simulink model "continuous_ex"  (R2022b)
settings: Solver=VariableStepAuto  StartTime=0.0  StopTime=10  FixedStep=0.1  RelTol=1e-3
libraries: simulink x1
settings Model: Creator=user  LastModifiedBy=user

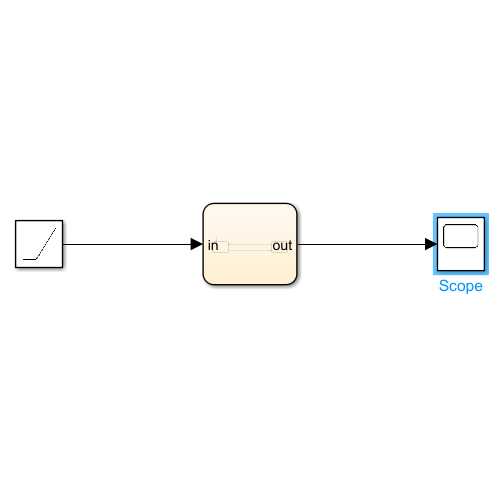
[thumbnail: Simulink's stored preview of the top-level diagram]
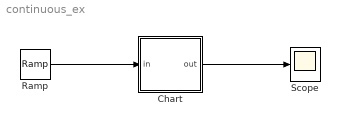
== system continuous_ex ==
  Chart : Stateflow chart  TreatAsAtomicUnit=on
  Ramp : simulink/Sources/Ramp  slope=1  start=0  InitialOutput=0
  Scope : Scope
  wires:
  Ramp/1 -> Chart/1(in)
  Chart/1(out) -> Scope/1

== stateflow chart continuous_ex/Chart ==
  settings: updateMethod=CONTINUOUS  sampleTime=1
  state POS
    en:
    out = in;
  state NEG
    out = -in;
  (default) -> POS
  NEG -> POS
  POS -> NEG
  data: in input; out output
